simulink model "ControladoresPlantilla"  (R2019b)
settings: Solver=ode45  StartTime=0.0  StopTime=500  RelTol=1e-6
values from neighbouring files (symbols this model uses):
  A = [(-((Ki*Kv*n^2)/(JLRa))-(Bm*n^2/(JL)))/Jt]    [EjercicioMotorCarga.m]
  B = [n*Ki/(JL*R*Jt),   -1/(JL*Jt)]    [EjercicioMotorCarga.m]
  C = [1 ... (first row only)    [EjercicioMotorCarga.m]
  D = [0 0 ... (first row only)    [EjercicioMotorCarga.m]
libraries: cstblocks x6
settings Model: Creator=B13  LastModifiedBy=l53

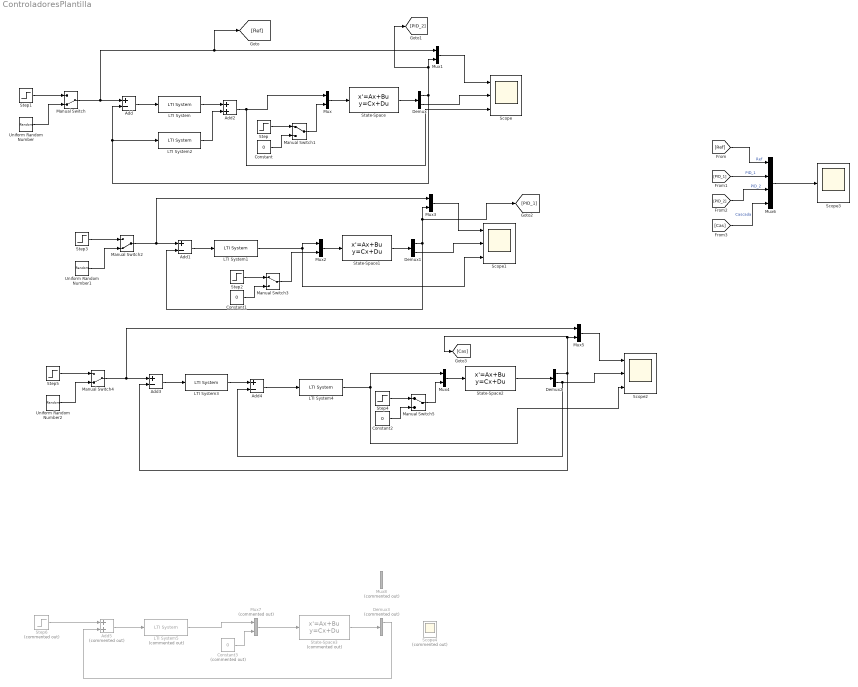
== system ControladoresPlantilla ==
  Add{,1,3..4} (4 alike) : Sum  Inputs=+-
  Add2 : Sum
  Add5 : Sum  Commented=on
  Constant : Constant  Value=0
  Constant1 : Constant  Value=0
  Constant2 : Constant  Value=0
  Constant3 : Constant  Commented=on  Value=0
  Demux : Demux  Outputs=2
  Demux1 : Demux  Outputs=2
  Demux2 : Demux  Outputs=2
  Demux3 : Demux  Commented=on  Outputs=2
  LTI System : cstblocks/LTI System  sys=Ca  IC=[]
  LTI System1 : cstblocks/LTI System  sys=Con  IC=[]
  LTI System2 : cstblocks/LTI System  sys=Cb  IC=[]
  LTI System3 : cstblocks/LTI System  sys=C2  IC=[]
  LTI System4 : cstblocks/LTI System  sys=C1  IC=[]
  LTI System5 : cstblocks/LTI System  Commented=on  sys=tf(1,[1 1])  IC=[]
  Manual Switch : ManualSwitch  CurrentSetting=0
  Manual Switch1 : ManualSwitch
  Manual Switch2 : ManualSwitch  CurrentSetting=0
  Manual Switch3 : ManualSwitch
  Manual Switch4 : ManualSwitch  CurrentSetting=0
  Manual Switch5 : ManualSwitch
  Mux{,1..5} (6 alike) : Mux  Inputs=2
  Mux6 : Mux
  Mux7 : Mux  Commented=on  Inputs=2
  Mux8 : Mux  Commented=on  Inputs=2
  Scope : Scope  NumInputPorts=3
  Scope1 : Scope  NumInputPorts=3
  Scope2 : Scope  NumInputPorts=3
  Scope3 : Scope
  Scope4 : Scope  Commented=on  NumInputPorts=3
  State-Space : StateSpace  A=A  B=B  C=C  D=D  InitialCondition=0
  State-Space1 : StateSpace  A=A  B=B  C=C  D=D  InitialCondition=0
  State-Space2 : StateSpace  A=A  B=B  C=C  D=D  InitialCondition=0
  State-Space3 : StateSpace  Commented=on  A=A  B=B  C=C  D=D  InitialCondition=0
  Step : Step  Time=20  SampleTime=0
  Step1 : Step  SampleTime=0
  Step2 : Step  Time=20  SampleTime=0
  Step3 : Step  SampleTime=0
  Step4 : Step  Time=20  SampleTime=0
  Step5 : Step  SampleTime=0
  Step6 : Step  Commented=on  SampleTime=0
  Uniform Random Number : UniformRandomNumber  SampleTime=50
  Uniform Random Number1 : UniformRandomNumber  SampleTime=50
  Uniform Random Number2 : UniformRandomNumber  SampleTime=50  VectorParams1D=off
  wires:
  State-Space/1 -> Demux/1
  Mux/1 -> State-Space/1
  Add/1 -> LTI System/1
  Demux/1 -> [PID_2], Mux1/2, LTI System2/1, Add/2
  Mux1/1 -> Scope/1
  Demux/2 -> Scope/2
  Manual Switch/1 -> [Ref], Mux1/1, Add/1
  Step1/1 -> Manual Switch/1
  Uniform Random Number/1 -> Manual Switch/2
  Step/1 -> Manual Switch1/1
  Manual Switch1/1 -> Mux/2
  Constant/1 -> Manual Switch1/2
  Constant1/1 -> Manual Switch3/2
  Manual Switch3/1 -> Mux2/2
  Step2/1 -> Manual Switch3/1
  Uniform Random Number1/1 -> Manual Switch2/2
  Step3/1 -> Manual Switch2/1
  Manual Switch2/1 -> Add1/1, Mux3/1
  Demux1/2 -> Scope1/2
  Mux3/1 -> Scope1/1
  Demux1/1 -> Add1/2, Mux3/2, [PID_1]
  Add1/1 -> LTI System1/1
  Mux2/1 -> State-Space1/1
  LTI System1/1 -> Scope1/3, Mux2/1
  State-Space1/1 -> Demux1/1
  LTI System/1 -> Add2/1
  Add2/1 -> Scope/3, Mux/1
  LTI System2/1 -> Add2/2
  LTI System3/1 -> Add4/1
  Constant2/1 -> Manual Switch5/2
  Manual Switch5/1 -> Mux4/2
  Step4/1 -> Manual Switch5/1
  Uniform Random Number2/1 -> Manual Switch4/2
  Step5/1 -> Manual Switch4/1
  Manual Switch4/1 -> Add3/1, Mux5/1
  Demux2/2 -> Add4/2, Scope2/2
  Mux5/1 -> Scope2/1
  Demux2/1 -> Add3/2, [Cas], Mux5/2
  Add3/1 -> LTI System3/1
  Mux4/1 -> State-Space2/1
  State-Space2/1 -> Demux2/1
  LTI System4/1 -> Scope2/3, Mux4/1
  Add4/1 -> LTI System4/1
  [Ref] -> Mux6/1  "Ref"
  [Cas] -> Mux6/4  "Cascada"
  [PID_2] -> Mux6/3  "PID_2"
  [PID_1] -> Mux6/2  "PID_1"
  Mux6/1 -> Scope3/1
  Step6/1 -> Add5/1
  Add5/1 -> LTI System5/1
  Mux7/1 -> State-Space3/1
  LTI System5/1 -> Mux7/1
  Constant3/1 -> Mux7/2
  State-Space3/1 -> Demux3/1
  Demux3/1 -> Add5/2
